simulink model "simulacao"  (R2020b)
settings: Solver=VariableStepAuto  StartTime=0.0  StopTime=10  RelTol=1e-3
values from neighbouring files (symbols this model uses):
  h = 0.1    [dados.m]
  M = 1    [dados.m]
  R = 1    [dados.m]
libraries: simulink x3
settings Model: Creator=lucas  LastModifiedBy=lucas

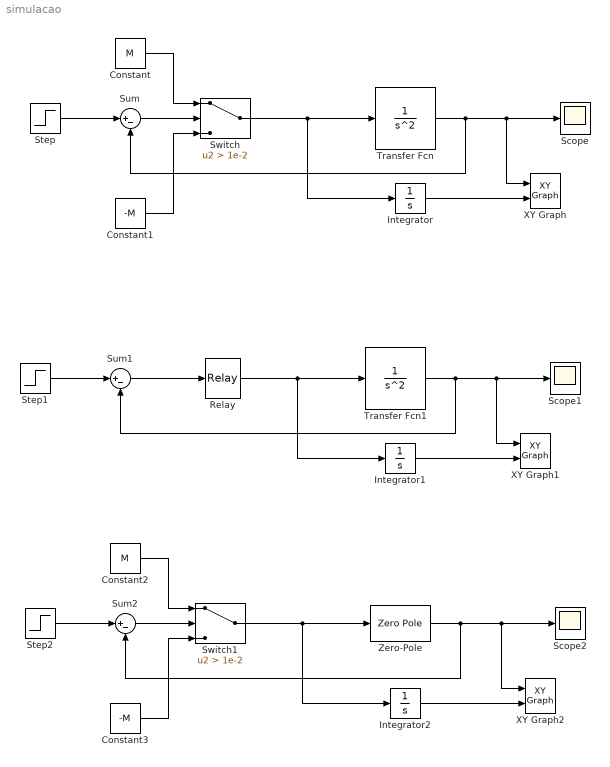
== system simulacao ==
  Constant : Constant  Value=M
  Constant1 : Constant  Value=-M
  Constant2 : Constant  Value=M
  Constant3 : Constant  Value=-M
  Integrator : Integrator
  Integrator1 : Integrator
  Integrator2 : Integrator
  Relay : Relay  OnSwitchValue=h  OffSwitchValue=-h  OnOutputValue=M  OffOutputValue=-M
  Scope : Scope
  Scope1 : Scope
  Scope2 : Scope
  Step : Step  After=R  SampleTime=0
  Step1 : Step  After=R  SampleTime=0
  Step2 : Step  After=R  SampleTime=0
  Sum : Sum  Inputs=|+-
  Sum1 : Sum  Inputs=|+-
  Sum2 : Sum  Inputs=|+-
  Switch : Switch  Criteria=u2 > Threshold  Threshold=1e-2
  Switch1 : Switch  Criteria=u2 > Threshold  Threshold=1e-2
  Transfer Fcn : TransferFcn  Denominator=[1 0 0 ]
  Transfer Fcn1 : TransferFcn  Denominator=[1 0 0 ]
  XY Graph : simulink/Sinks/XY Graph  xmin=-4*R  xmax=4*R  ymin=-7*R  ymax=7*R  st=-1
  XY Graph1 : simulink/Sinks/XY Graph  xmin=-4*R  xmax=4*R  ymin=-7*R  ymax=7*R  st=-1
  XY Graph2 : simulink/Sinks/XY Graph  xmin=-4*R  xmax=4*R  ymin=-7*R  ymax=7*R  st=-1
  Zero-Pole : ZeroPole  Zeros=[]  Poles=[0 -1]
  wires:
  Switch/1 -> Integrator/1, Transfer Fcn/1
  Step/1 -> Sum/1
  Sum/1 -> Switch/2
  Transfer Fcn/1 -> Scope/1, XY Graph/1, Sum/2
  Integrator/1 -> XY Graph/2
  Constant/1 -> Switch/1
  Constant1/1 -> Switch/3
  Relay/1 -> Integrator1/1, Transfer Fcn1/1
  Sum1/1 -> Relay/1
  Integrator1/1 -> XY Graph1/2
  Transfer Fcn1/1 -> Scope1/1, XY Graph1/1, Sum1/2
  Step1/1 -> Sum1/1
  Constant3/1 -> Switch1/3
  Switch1/1 -> Zero-Pole/1, Integrator2/1
  Constant2/1 -> Switch1/1
  Sum2/1 -> Switch1/2
  Integrator2/1 -> XY Graph2/2
  Zero-Pole/1 -> Scope2/1, XY Graph2/1, Sum2/2
  Step2/1 -> Sum2/1
